simulink model "Sector_Popov_test"  (Simulink 7.3)
settings: Solver=ode45  StartTime=0.0  StopTime=10.0  RelTol=1e-3
settings Model: Creator=MD710  LastModifiedBy=MD710
settings DebuggingCC: SaveWithParameterizedLinksMsg=none  SolverPrmCheckMsg=none  MultiTaskDSMMsg=warning  MultiTaskCondExecSysMsg=none  FcnCallInpInsideContextMsg=Enable All  StrictBusMsg=None
settings HardwareCC: TargetHWDeviceType=32-bit Generic
settings RTWCC: IncludeERTFirstTime=on
settings GRTTargetCC: TargetFcnLib=ansi_tfl_tmw.mat

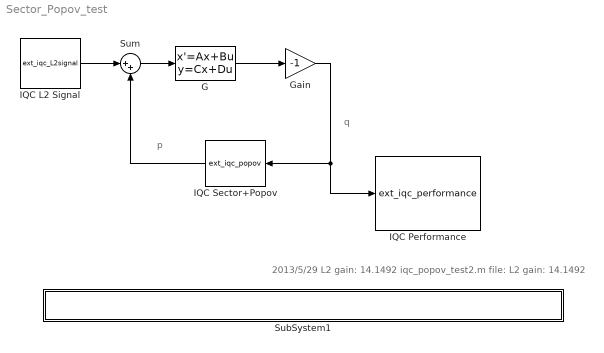
== system Sector_Popov_test ==
  note: q
  note: p
  note: 2013/5/29 L2 gain: 14.1492
      | iqc_popov_test2.m file: L2 gain: 14.1492
  G : StateSpace  A=[-0.1 -1;1 0]  B=[1;0]  C=[1 1]  D=0
  Gain : Gain  Gain=-1
  IQC L2 Signal : M-S-Function  FunctionName=ext_iqc_L2signal  Parameters=sig_size,sam_time,sig_type,tru_time,sig_amp,sig_fre,user_cus  mask(IQC L2 signal(ver:0.1)){sig_size=1, sam_time=0, sig_type=Step, tru_time=10, sig_amp=1, sig_fre=1, user_cus='2*exp(3*t)'}
      mask prompts: sig_size "Signal Dimension:(Default: 1)"; sam_time "Sample Time:(Default: 0)"; sig_type "Signal Type:"; tru_time "Truncation Time:"; sig_amp "Maximum Amplitude:"; sig_fre "Frequency:"; user_cus "Custom:"
      mask help:
      | Important:
      | In IQC procedure step (as commond iqc_gain_tbx, the task is get
      | L2 gain value), regardless of the user to choose which option (ex sine...),
      | here regarded as generalized L2 signal.
      mask StyleString: edit,edit,popup(Step|Square wave|Sine wave|Custom|Random|External),edit,edit,edit,edit
      mask CallbackString: ||iqc_block_cho(gcb,'L2signal_type')||||
      mask TabNameString: Generalized Parameters,Generalized Parameters,Simulink Parameters,Simulink Parameters,Simulink Parameters,Simulink Parameters,Simulink Parameters
      mask Display: plot(0:0.1:10,[sin(0:0.1:6.2) zeros(1,38)])
  IQC Performance : M-S-Function  FunctionName=ext_iqc_performance  Parameters=imp_met,save_lin_com,isiqcbode,fre_ran,uselmitool,lmi_par  mask(IQC Performance(ver:0.1)){imp_met=Only Calculation, save_lin_com=off, isiqcbode=off, fre_ran='', uselmitool=lmilab, lmi_par=''}
      mask prompts: imp_met "Implementation Methods"; save_lin_com "Save the Linear File and Command File"; isiqcbode "Display IQC Bode Figure"; fre_ran "Frequency Range:(Default: empty)"; uselmitool "LMI Tool:"; lmi_par "Parameter:(if empty use define)"
      mask help:
      | Important:
      | In IQC toolbox calculate step (as commond iqc_gain_tbx, the task is get
      | L2 gain value), regardless of the user to connect any signal input(Even if
      | not a signal), here regarded as generalized L2 signal.
      |
      | Example 1: setlmioptions('',[0 200 0 0 777])
      | the block parameter is
      | LMI Tool: lmilab
      | Parameter:
      |        [0 200 0 0 777]
      |
      | Example 2: setlmioptions('yalmip','solver','sdpt3','verbose',1)
      | the block parameter is
      | LMI Tool: yalmip
      | Parameter:
      |        {'solver',sdpt3','verbose',1}
      mask Help:
      | <a href="matlab:doc abst_init_iqc;">abst_init_iqc</a>
      | <a href="matlab:doc setlmioptions;">setlmioptions</a>
      | <a href="matlab:doc iqc_gain_tbx;">iqc_gain_tbx</a>
      mask StyleString: popup(Calculation and Simulation|Only Calculation|Only Simulation),checkbox,checkbox,edit,popup(lmilab|yalmip),edit
      mask CallbackString: iqc_block_cho(gcb,'performance_imp')||iqc_block_cho(gcb,'performance_bodefre')|||
      mask TabNameString: Parameter,Parameter,Parameter,Parameter,LMI Parameter,LMI Parameter
      mask Display: fprintf('In -> Out \n performance \n L2 gain:\n%4.4f',14.1492);
  IQC Sector+Popov : M-S-Function  FunctionName=ext_iqc_popov  Parameters=low_sec,upp_sec,out_var  mask(IQC Sector+Popov(ver:0.1)){low_sec=0, upp_sec=1, out_var=''}
      mask prompts: low_sec "Low Sector Bound:(Default: 0)"; upp_sec "Upper Sector Bound:(Default: 1)"; out_var "Output Variable:(Default: empty)"
      mask help:
      | Example: [w,X,Y]=iqc_popov(v,alpha,beta)
      | Low Sector Bound:
      |                alpha
      | Upper Sector Bound:
      |                beta
      | Output Variable:
      |                {'X','Y'}
      mask Help: eval('doc iqc_popov')
      mask Display: plot(0,0,100,100,[100,-0],[54,54],[50,50],[0,100],[66,32],[100,0],[-0,100],[37,71],[20,-0],[0,32],[33,13],[5,41],[40,28],[24,46],[47,42],[44,51],[65,57],[60,73],[78,63],[64,90],[95,77],[69,100],[91,85,82,78,77,75,74,66,61,56,54,50,48,45,43,42,40,38,35,31,27,24,21,17,14,11,10,8,7],[96,96,93,90,82,76,71,66,66,63,60,54,51,49,46,42,38,34,32,32,32,32,32,31,29,27,24,18,13]);
  SubSystem1 : Subsystem  mask{filename=iqc_popov_test2.m}
      mask init:
      | x_dir=which(filename);
      | x=x_dir;
      settings: OpenFcn=|
      | x_dir=which('iqc_popov_test2.m');
      | x=x_dir;
      | edit(x);
      mask Display: disp(['MATLAB file: ' x]);
  Sum : Sum  Inputs=|++
  wires:
  G/1 -> Gain/1
  Sum/1 -> G/1
  IQC L2 Signal/1 -> Sum/1
  Gain/1 -> IQC Performance/1, IQC Sector+Popov/1
  IQC Sector+Popov/1 -> Sum/2

== system Sector_Popov_test/SubSystem1 ==
